simulink model "simBiorreactor_OD"  (R2020b)
settings: Solver=ode45  StartTime=0.0  StopTime=1000  MaxStep=1  RelTol=1e-3  AbsTol=1e-6
undefined symbols (not defined in the file or in its folder): p
settings Model: Creator=nobel  LastModifiedBy=nobel

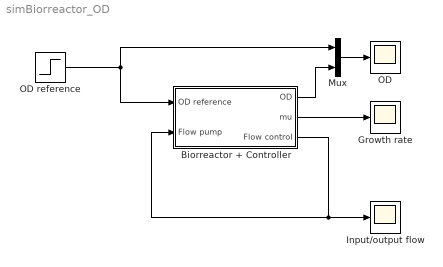
== system simBiorreactor_OD ==
  Biorreactor + Controller : Subsystem
  Growth rate : Scope
  Input/output flow : Scope
  Mux : Mux  Inputs=2
  OD : Scope
  OD reference : Step  Time=500  Before=1  After=2  SampleTime=0
  wires:
  OD reference/1 -> Mux/1, Biorreactor + Controller/1(OD reference)
  Biorreactor + Controller/2(mu) -> Growth rate/1
  Biorreactor + Controller/3(Flow control) -> Input/output flow/1, Biorreactor + Controller/2(Flow pump)
  Mux/1 -> OD/1
  Biorreactor + Controller/1(OD) -> Mux/2

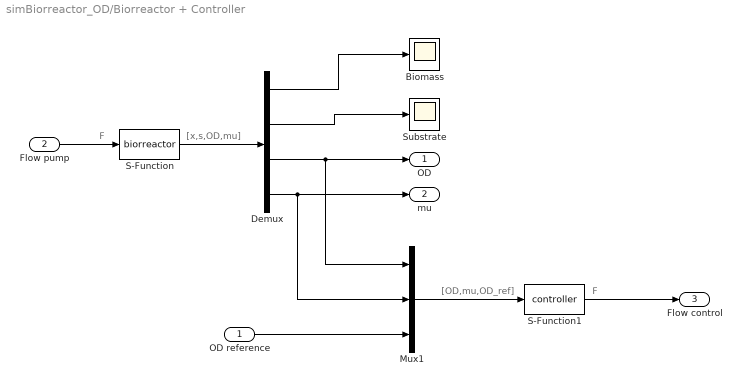
== system simBiorreactor_OD/Biorreactor + Controller ==
  note: [OD,mu,OD_ref]
  note: F
  note: [x,s,OD,mu]
  note: F
  OD reference : Inport
  Flow pump : Inport  Port=2
  Biomass : Scope
  Demux : Demux
  Mux1 : Mux  Inputs=3
  S-Function : S-Function  FunctionName=biorreactor  Parameters=[0.1 16],p  SFunctionDeploymentMode=off  EnableBusSupport=off
  S-Function1 : S-Function  FunctionName=controller  Parameters=p  SFunctionDeploymentMode=off  EnableBusSupport=off
  Substrate : Scope
  OD : Outport
  mu : Outport  Port=2
  Flow control : Outport  Port=3
  wires:
  Demux/4 -> Mux1/2, mu/1
  Demux/3 -> Mux1/1, OD/1
  OD reference/1 -> Mux1/3
  S-Function/1 -> Demux/1
  Demux/2 -> Substrate/1
  Mux1/1 -> S-Function1/1
  S-Function1/1 -> Flow control/1
  Demux/1 -> Biomass/1
  Flow pump/1 -> S-Function/1
